simulink model "Atomic_Subsystem"  (R2020b)
settings: Solver=VariableStepAuto  StartTime=0.0  StopTime=10.0  RelTol=1e-3
settings Model: Creator=shweta  LastModifiedBy=shweta
settings DataIOCC: SaveOutput=off  SaveTime=off

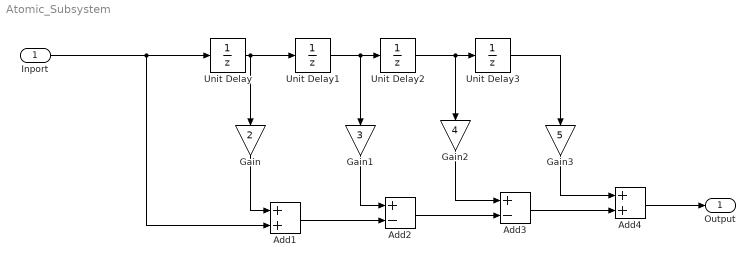
== system Atomic_Subsystem ==
  Inport : Inport  OutDataTypeStr=double  PortDimensions=1  SampleTime=0
  Add1 : Sum
  Add2 : Sum  Inputs=+-
  Add3 : Sum  Inputs=+-
  Add4 : Sum
  Gain : Gain  Gain=2
  Gain1 : Gain  Gain=3
  Gain2 : Gain  Gain=4
  Gain3 : Gain  Gain=5
  Unit Delay{,1..3} (4 alike) : UnitDelay  SampleTime=-1  HasFrameUpgradeWarning=on
  Output : Outport  OutDataTypeStr=double  PortDimensions=1  SampleTime=0
  wires:
  Add4/1 -> Output/1
  Add3/1 -> Add4/2
  Gain2/1 -> Add3/1
  Add1/1 -> Add2/2
  Gain/1 -> Add1/1
  Unit Delay/1 -> Gain/1, Unit Delay1/1
  Unit Delay2/1 -> Unit Delay3/1, Gain2/1
  Unit Delay1/1 -> Unit Delay2/1, Gain1/1
  Add2/1 -> Add3/2
  Gain3/1 -> Add4/1
  Unit Delay3/1 -> Gain3/1
  Gain1/1 -> Add2/1
  Inport/1 -> Unit Delay/1, Add1/2
